simulink model "simulatore"  (R2016a)
settings: Solver=VariableStepAuto  StartTime=0.0  StopTime=100  RelTol=1e-3
libraries: X8_lib x1
settings Model: Creator=andreanv  LastModifiedBy=andreanv

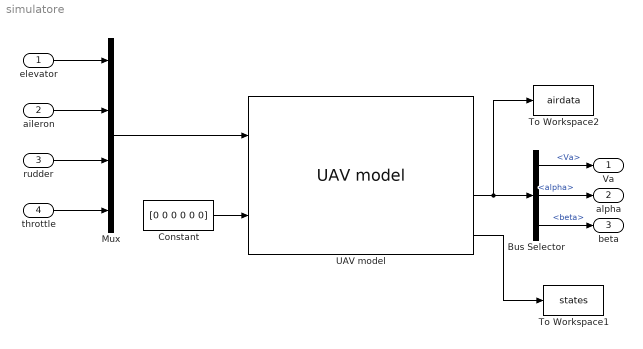
== system simulatore ==
  elevator : Inport
  aileron : Inport  Port=2
  rudder : Inport  Port=3
  throttle : Inport  Port=4
  Bus Selector : BusSelector  OutputSignals=Va,alpha,beta
  Constant : Constant  Value=[0 0 0 0 0 0]
  Mux : Mux
  To Workspace1 : ToWorkspace  VariableName=states  SaveFormat=Timeseries  SampleTime=-1
  To Workspace2 : ToWorkspace  VariableName=airdata  SaveFormat=Timeseries  SampleTime=-1
  UAV model : X8_lib/UAV model  param=param  pos0=[0,0,-100]  quat0=[1,0,0,0]  vel0=[0,0,0]  rate0=[0,0,0]  servoR_pos0=0  servoR_vel0=0  servoL_pos0=0  servoL_vel0=0  motor_speed0=0
  Va : Outport
  alpha : Outport  Port=2
  beta : Outport  Port=3
  wires:
  aileron/1 -> Mux/2
  elevator/1 -> Mux/1
  rudder/1 -> Mux/3
  throttle/1 -> Mux/4
  Mux/1 -> UAV model/1
  Constant/1 -> UAV model/2
  UAV model/3 -> To Workspace2/1, Bus Selector/1
  Bus Selector/1 -> Va/1  "<Va>"
  Bus Selector/2 -> alpha/1  "<alpha>"
  Bus Selector/3 -> beta/1  "<beta>"
  UAV model/4 -> To Workspace1/1
